simulink model "KeyEventGenerator"  (R2016b)
settings: Solver=VariableStepAuto  StartTime=0.0  StopTime=10.0  RelTol=1e-3
settings Model: Creator=lucadelaat  LastModifiedBy=lucadelaat
settings DataIOCC: SaveOutput=off  SaveTime=off

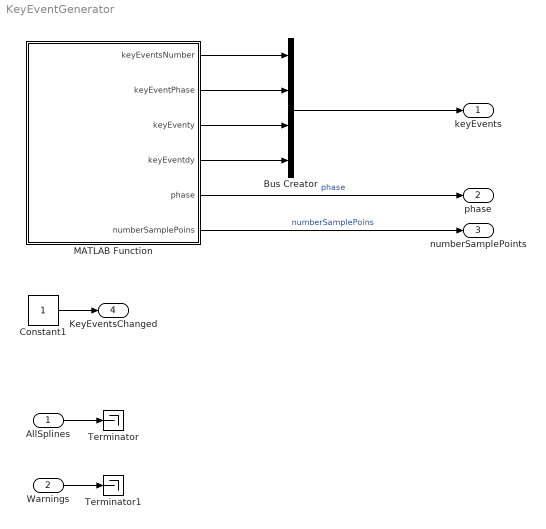
== system KeyEventGenerator ==
  AllSplines : Inport
  Warnings : Inport  Port=2
  Bus Creator : BusCreator  Inputs=4
  Constant1 : Constant
  MATLAB Function : MATLAB Function  TreatAsAtomicUnit=on
  Terminator : Terminator
  Terminator1 : Terminator
  keyEvents : Outport  OutDataTypeStr=Bus: slBus1  SampleTime=[0,1]
  phase : Outport  Port=2  OutDataTypeStr=double  PortDimensions=1001  SampleTime=[0,1]
  numberSamplePoints : Outport  Port=3  OutDataTypeStr=double  PortDimensions=1  SampleTime=[0,1]
  KeyEventsChanged : Outport  Port=4  OutDataTypeStr=double  PortDimensions=1
  wires:
  Constant1/1 -> KeyEventsChanged/1
  MATLAB Function/6(numberSamplePoins) -> numberSamplePoints/1  "numberSamplePoins"
  MATLAB Function/5(phase) -> phase/1  "phase"
  Bus Creator/1 -> keyEvents/1
  MATLAB Function/1(keyEventsNumber) -> Bus Creator/1
  MATLAB Function/2(keyEventPhase) -> Bus Creator/2
  MATLAB Function/3(keyEventy) -> Bus Creator/3
  MATLAB Function/4(keyEventdy) -> Bus Creator/4
  AllSplines/1 -> Terminator/1
  Warnings/1 -> Terminator1/1

== matlab function KeyEventGenerator/MATLAB Function ==
  data: keyEventsNumber output; keyEventPhase output; keyEventy output; keyEventdy output; phase output; numberSamplePoins output
function [keyEventsNumber, keyEventPhase,keyEventy,keyEventdy, phase, numberSamplePoins] = fcn()

keyEventPhase = [0, 20, 40, 60, 80, 100];
keyEventy = [0, 40, 30, -10, -10, 0];
keyEventdy = [0,-1,-1,0,1,0];

phase = (0:0.1:100)';

numberSamplePoins = 100;

keyEventsNumber = length(keyEventPhase);
end
